simulink model "motorLearning"  (R2016b)
settings: Solver=ode1  StartTime=0.0  StopTime=inf  FixedStep=0.01  RelTol=1e-3
undefined symbols (not defined in the file or in its folder): serial
libraries: instrumentlib x2, simulink x1, dspfdesign x1
settings Model: Creator=admin  LastModifiedBy=admin

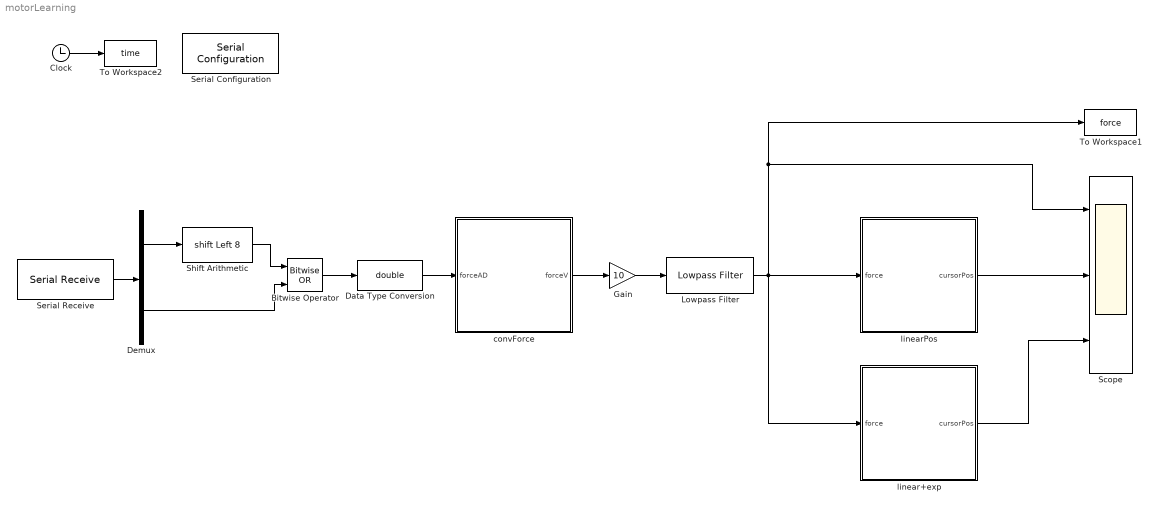
== system motorLearning ==
  Bitwise Operator : simulink/Logic and Bit Operations/Bitwise Operator  logicop=OR  UseBitMask=off  NumInputPorts=2  BitMask=bin2dec('11011001')  BitMaskRealWorld=Stored Integer
  Clock : Clock
  Data Type Conversion : DataTypeConversion  OutDataTypeStr=double
  Demux : Demux  Outputs=2
  Gain : Gain  Gain=10
  Lowpass Filter : dspfdesign/Lowpass Filter  FilterType=IIR  DesignForMinimumOrder=on  FilterOrder=50  PassbandFrequency=1  StopbandFrequency=20  PassbandRipple=0.1  StopbandAttenuation=20  InheritSampleRate=off  SampleRate=100  SimulateUsing=Interpreted execution  roundingMode=Floor  coeffsDataTypeStr=fixdt(1,16)
  Scope : Scope  NumInputPorts=3
  Serial Configuration : instrumentlib/Serial Configuration  Priority=-200000  ComPortMenu=COM6  ComPort=COM6  ObjConstructor=serial('COM6');  BaudRate=38400  DataBits=8  Parity=none  StopBits=1  FlowControl=none  Timeout=10  ByteOrder=LittleEndian
  Serial Receive : instrumentlib/Serial Receive  ComPortMenu=COM6  ComPort=COM6  ObjConstructor=serial('COM6');  Header=$  Terminator=!  DataSize="[1  2]"  DataType=uint8  EnableBlockingMode=on  ActionDataUnavailable=Output last received value  CustomValue=0  SampleTime=0.01
  Shift Arithmetic : ArithShift  BitShiftNumber=8  BitShiftDirection=Left
  To Workspace1 : ToWorkspace  VariableName=force  SampleTime=-1
      settings: Save2DSignal=2-D array (concatenate along first dimension)
  To Workspace2 : ToWorkspace  VariableName=time  SampleTime=-1
      settings: Save2DSignal=2-D array (concatenate along first dimension)
  convForce : MATLAB Function  TreatAsAtomicUnit=on
  linear+exp : MATLAB Function  TreatAsAtomicUnit=on
  linearPos : MATLAB Function  TreatAsAtomicUnit=on
  wires:
  Serial Receive/1 -> Demux/1
  Demux/1 -> Shift Arithmetic/1
  Shift Arithmetic/1 -> Bitwise Operator/1
  Demux/2 -> Bitwise Operator/2
  Bitwise Operator/1 -> Data Type Conversion/1
  Data Type Conversion/1 -> convForce/1(forceAD)
  Lowpass Filter/1 -> linear+exp/1(force), linearPos/1(force), To Workspace1/1, Scope/1
  Clock/1 -> To Workspace2/1
  convForce/1(forceV) -> Gain/1
  Gain/1 -> Lowpass Filter/1
  linear+exp/1(cursorPos) -> Scope/3
  linearPos/1(cursorPos) -> Scope/2

== matlab function motorLearning/convForce ==
  data: forceAD input; forceV output
function forceV = convForce(forceAD)

forceV = (forceAD*5) / (1023);

== matlab function motorLearning/linear+exp ==
  data: force input; cursorPos output
function cursorPos = convertPosition(force)

minForce = 0;
maxForce = 5;

minScreen = 10;
maxScreen = 1536;

p = polyfit([minForce,maxForce],[minScreen,maxScreen],1);

if(force <= 2)
    cursorPos = p(1)*force + p(2);
else
    x = exp(force);    
    xmin = exp(2);
    xmax = exp(maxForce);
    ymin=maxScreen/2;
    ymax=maxScreen;
    cursorPos = ((x-xmin).*(ymax-ymin) ./ (xmax-xmin)) + ymin;    
end

== matlab function motorLearning/linearPos ==
  data: force input; cursorPos output
function cursorPos = convertPosition(force)

minForce = 0;
maxForce = 5;

minScreen = 10;
maxScreen = 1536;

p = polyfit([minForce,maxForce],[minScreen,maxScreen],1);

cursorPos = p(1)*force + p(2);
   
end
